simulink model "problem_4_model"  (R2020b)
settings: Solver=VariableStepAuto  StartTime=0.0  StopTime=20  RelTol=1e-3
settings Model: Creator=Arvind Hishikar  LastModifiedBy=Arvind Hishikar

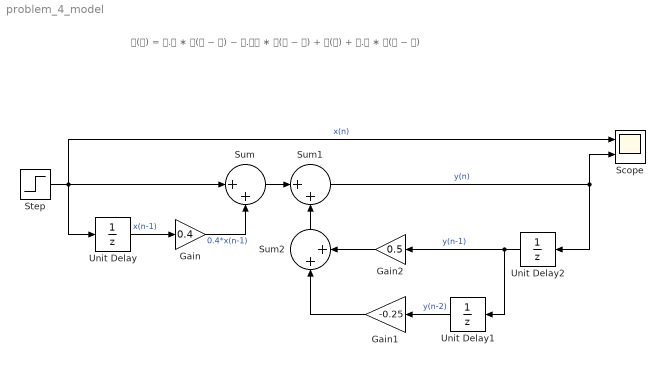
== system problem_4_model ==
  note: 𝐲(𝐧) = 𝟎.𝟓 ∗ 𝐲(𝐧 − 𝟏) − 𝟎.𝟐𝟓 ∗ 𝐲(𝐧 − 𝟐) + 𝐱(𝐧) + 𝟎.𝟒 ∗ 𝐱(𝐧 − 𝟏)
  Gain : Gain  Gain=0.4
  Gain1 : Gain  Gain=-0.25
  Gain2 : Gain  Gain=0.5
  Scope : Scope  NumInputPorts=2
  Step : Step  SampleTime=0
  Sum : Sum  Inputs=|++
  Sum1 : Sum  Inputs=|++
  Sum2 : Sum  Inputs=|++
  Unit Delay : UnitDelay  SampleTime=-1  HasFrameUpgradeWarning=on
  Unit Delay1 : UnitDelay  SampleTime=-1  HasFrameUpgradeWarning=on
  Unit Delay2 : UnitDelay  SampleTime=-1  HasFrameUpgradeWarning=on
  wires:
  Unit Delay/1 -> Gain/1  "x(n-1)"
  Step/1 -> Unit Delay/1, Scope/1, Sum/1  "x(n)"
  Gain/1 -> Sum/2  "0.4*x(n-1)"
  Sum/1 -> Sum1/1
  Unit Delay2/1 -> Gain2/1, Unit Delay1/1  "y(n-1)"
  Sum1/1 -> Unit Delay2/1, Scope/2  "y(n)"
  Unit Delay1/1 -> Gain1/1  "y(n-2)"
  Gain2/1 -> Sum2/2
  Gain1/1 -> Sum2/1
  Sum2/1 -> Sum1/2
